simulink model "DriverCon"  (R2020a)
settings: Solver=VariableStepAuto  StartTime=0.0  StopTime=10.0  RelTol=1e-3
model workspace (MAT data in the model file):
  VEH.Mass = 330
  VEH.StaticNormalFrontLoad.FR = 74.25
  VEH.StaticNormalFrontLoad.FL = 74.25
  VEH.StaticNormalRearLoad.RR = 90.75
  VEH.StaticNormalRearLoad.RL = 90.75
  VEH.WheelBase = 1.54
  VEH.FrontAxlePositionfromCG = 0.847
  VEH.RearAxlePositionfromCG = 0.693
  VEH.HeightCG = 0.283
  VEH.FrontalArea = 2.11
  VEH.DragCoefficient = 0.33
  VEH.NumberOfWheelsPerAxle = 2
  VEH.Thread.FR = 1.705
  VEH.Thread.RR = 1.705
  VEH.PitchMomentInertia = 206
  VEH.RollMomentInertia = 206.613792
  VEH.YawMomentInertia = 206.613792
  VEH.SteeringRatio = 5.2
  VEH.TrackWidth = 1.2
  VEH.SprungMass = 290
  VEH.InitialLongPosition = 0
  VEH.InitialLatPosition = 0
  VEH.InitialVertPosition = 0
  VEH.InitialRollAngle = 0
  VEH.InitialPitchAngle = 0
  VEH.InitialYawAngle = 0
  VEH.InitialLongVel = 0
  VEH.InitialLatVel = 0
  VEH.InitialVertVel = 0
  VEH.InitialRollRate = 0
  VEH.InitialPitchRate = 0
  VEH.InitialYawRate = 0
libraries: vehdynlibdriver x1
settings Model: Creator=Administrator  LastModifiedBy=Administrator

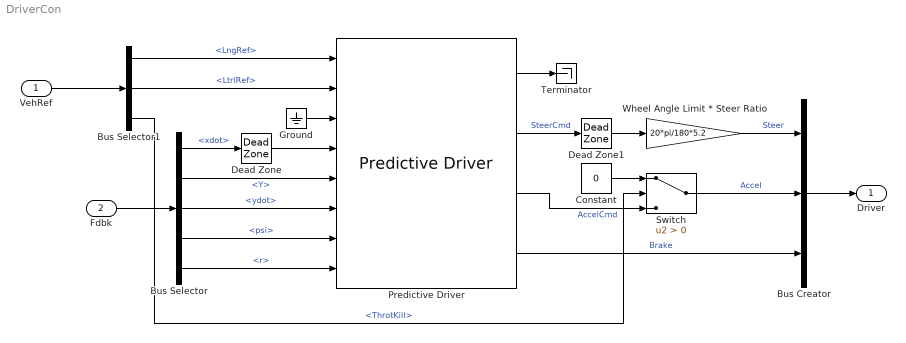
== system DriverCon ==
  VehRef : Inport
  Fdbk : Inport  Port=2
  Bus Creator : BusCreator  Inputs=3
  Bus Selector : BusSelector  OutputSignals=Body.xdot,Body.Y,Body.ydot,Body.psi,Body.r
  Bus Selector1 : BusSelector  OutputSignals=LngRef,LtrlRef,ThrotKill
  Constant : Constant  Value=0
  Dead Zone : DeadZone  ZeroCross=off  SaturateOnIntegerOverflow=on
  Dead Zone1 : DeadZone  LowerValue=-1e-2  UpperValue=1e-2  ZeroCross=off  SaturateOnIntegerOverflow=on
  Ground : Ground
  Predictive Driver : vehdynlibdriver/Predictive Driver  extAccelOvr=off  extDecelOvr=off  extAccelHld=off  extDecelHld=off  extAccelZero=off  extDecelZero=off  extSteerOvr=off  extSteerHld=off  extSteerZero=off  cntrlType=PI  shftType=None  velUnits=m/s  gearOut=off  steerOut=off  Kp=10  Ki=5  Kff=.1  Kg=0  VehVelVec=[0 100]  KffVec=[.1 .1]  KpVec=[10 10]  KiVec=[5 5]  KgVec=[0 0]  vnom=35  Kaw=1  tauerr=.01  a=VEH.FrontAxlePositionfromCG  b=VEH.RearAxlePositionfromCG  m=VEH.Mass  I=VEH.YawMomentInertia  Cy_f=11459  Cy_r=11459  theta=30*pi/180  Ksteer=18  tau=0.03  L=1.0  Kpt=3000  aR=200  bR=2.5  cR=.5  g=9.81  GearInit=0  tShift=.1  pdlVec=[0.1 0.4 0.5 0.9]  upShftTbl=[-1 12.9375 26.4375 39.9375 51.18749999999999 62.4375 72.84375 83.25;-1 16.3125 29.8125 43.3125 54.5624 65.8125 76.78125 87.75;-1 19.6875 33.1875 46.68749999999999 57.9375 69.1875 80.71875 92.25;-1 33 52.5 77.25 100.5 138.75 161.875 185]  dwnShftTbl=[-1 12.9375 26.4375 39.9375 51.18749999999999 62.4375 72.84375 83.25;-1 16.3125 29.8125 43.3125 54.5624 65.8125 76.78125 87.75;-1 19.6875 33.1875 46.68749999999999 57.9375 69.1875 80.71875 92.25;-1 33 52.5 77.25 100.5 138.75 161.875 185]  tClutch=.5  tRev=.5  tPark=120  aMode=2  UpGearVec="[0  1  2  3  4  5  6  7]"  DownGearVec="[1  2  3  4  5  6  7  8]"
      settings: SourceProductBaseCode=VE
  Switch : Switch  Criteria=u2 > Threshold
  Terminator : Terminator
  Wheel Angle Limit * Steer Ratio : Gain  Gain=20*pi/180*5.2
  Driver : Outport  VectorParamsAs1DForOutWhenUnconnected=off
  wires:
  Ground/1 -> Predictive Driver/3
  Constant/1 -> Switch/1
  Predictive Driver/4 -> Bus Creator/3  "Brake"
  VehRef/1 -> Bus Selector1/1
  Predictive Driver/3 -> Switch/3  "AccelCmd"
  Bus Selector/3 -> Predictive Driver/6  "<ydot>"
  Dead Zone1/1 -> Wheel Angle Limit * Steer Ratio/1
  Dead Zone/1 -> Predictive Driver/4
  Bus Creator/1 -> Driver/1
  Predictive Driver/1 -> Terminator/1
  Bus Selector/5 -> Predictive Driver/8  "<r>"
  Wheel Angle Limit * Steer Ratio/1 -> Bus Creator/1  "Steer"
  Bus Selector/2 -> Predictive Driver/5  "<Y>"
  Predictive Driver/2 -> Dead Zone1/1  "SteerCmd"
  Bus Selector/1 -> Dead Zone/1  "<xdot>"
  Bus Selector/4 -> Predictive Driver/7  "<psi>"
  Bus Selector1/3 -> Switch/2  "<ThrotKill>"
  Bus Selector1/1 -> Predictive Driver/1  "<LngRef>"
  Switch/1 -> Bus Creator/2  "Accel"
  Fdbk/1 -> Bus Selector/1
  Bus Selector1/2 -> Predictive Driver/2  "<LtrlRef>"
